simulink model "Dynamic_RR"  (R2019b)
settings: Solver=VariableStepAuto  StartTime=0.0  StopTime=30  FixedStep=1e-2  RelTol=1e-3
undefined symbols (not defined in the file): pi_hat_0, pi_param, qInitial_0
settings Model: Creator=Stefano  LastModifiedBy=Stefano

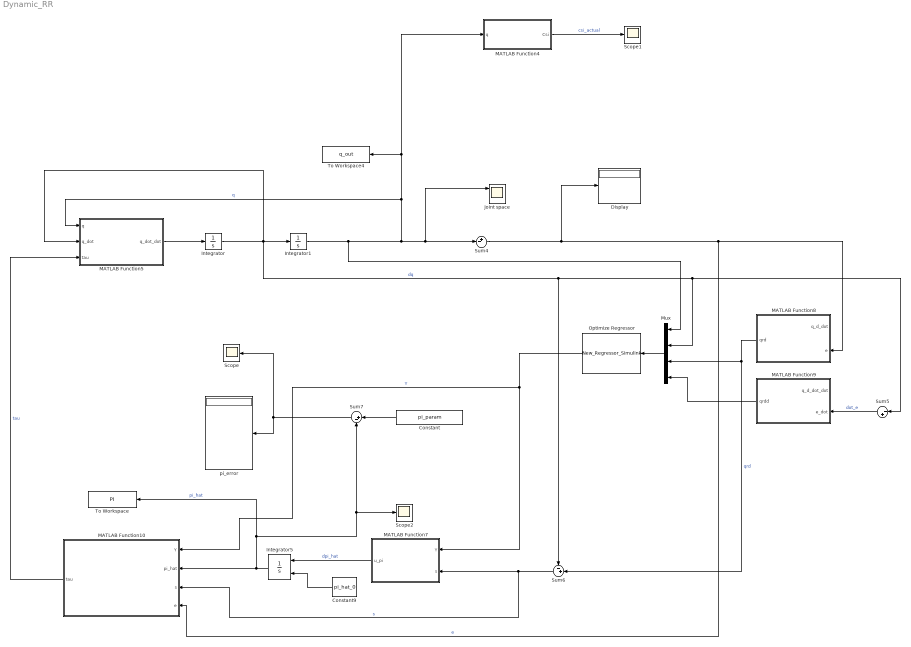
== system Dynamic_RR ==
  Constant : Constant  Value=pi_param
  Constant9 : Constant  Value=pi_hat_0
  Display : Display
  Integrator : Integrator  InitialCondition=qInitial_0
  Integrator1 : Integrator  InitialCondition=[0,0]'
  Integrator5 : Integrator  InitialConditionSource=external
  Joint space : Scope  NumInputPorts=2
  MATLAB Function10 : MATLAB Function  TreatAsAtomicUnit=on
  MATLAB Function4 : MATLAB Function  TreatAsAtomicUnit=on
  MATLAB Function5 : MATLAB Function  TreatAsAtomicUnit=on
  MATLAB Function7 : MATLAB Function  TreatAsAtomicUnit=on
  MATLAB Function8 : MATLAB Function  TreatAsAtomicUnit=on
  MATLAB Function9 : MATLAB Function  TreatAsAtomicUnit=on
  Mux : Mux
  "Optimize Regressor " : MATLABFcn  MATLABFcn=New_Regressor_Simulink  OutputDimensions=[2,6]  Output1D=off
  Scope : Scope
  Scope1 : Scope
  Scope2 : Scope
  Sum4 : Sum  Inputs=+-|
  Sum5 : Sum  Inputs=|-+
  Sum6 : Sum  Inputs=-+|
  Sum7 : Sum  Inputs=|+-
  To Workspace : ToWorkspace  VariableName=PI  SaveFormat=Timeseries  SampleTime=-1
  To Workspace4 : ToWorkspace  VariableName=q_out  SaveFormat=Timeseries  SampleTime=-1
  pi_error : Display
  wires:
  Sum6/1 -> MATLAB Function10/3(s), MATLAB Function7/2(s)  "s"
  Sum4/1 -> Display/1, MATLAB Function10/4(e), MATLAB Function8/2(e)  "e"
  Sum5/1 -> MATLAB Function9/2(e_dot)  "dot_e"
  MATLAB Function7/1(u_pi) -> Integrator5/1  "dpi_hat"
  Integrator5/1 -> MATLAB Function10/2(pi_hat), To Workspace/1, Scope2/1, Sum7/2  "pi_hat"
  Integrator/1 -> MATLAB Function5/2(q_dot), Sum5/1, Mux/2, Sum6/1, Integrator1/1  "dq"
  Constant9/1 -> Integrator5/2
  MATLAB Function8/1(qrd) -> Sum6/2, Mux/3  "qrd"
  Mux/1 -> "Optimize Regressor "/1
  MATLAB Function9/1(qrdd) -> Mux/4
  Constant/1 -> Sum7/1
  Sum7/1 -> Scope/1, pi_error/1
  Integrator1/1 -> Mux/1, To Workspace4/1, MATLAB Function4/1(q), MATLAB Function5/1(q), Joint space/1, Sum4/2  "q"
  "Optimize Regressor "/1 -> MATLAB Function10/1(Y), MATLAB Function7/1(Y)  "Y"
  MATLAB Function10/1(tau) -> MATLAB Function5/3(tau)  "tau"
  MATLAB Function5/1(q_dot_dot) -> Integrator/1
  ? -> Joint space/2, Sum4/1
  ? -> MATLAB Function8/1(q_d_dot), Sum5/2
  ? -> MATLAB Function9/1(q_d_dot_dot)
  MATLAB Function4/1(Csi) -> Scope1/1  "csi_actual"

== matlab function Dynamic_RR/MATLAB Function5 ==
  data: q input; q_dot_dot output; q_dot input; tau input
function q_dot_dot = Forward_Dynamics(q,q_dot,tau)

m1 = 1;
m2 = 1;

l1=1;
l2=1;

r1=l1/2;
r2=l2/2;


Izz1 = (1/12)*m1*l1^2;
Izz2 = (1/12)*m2*l2^2;



Alpha = Izz1 + Izz2 + m1*(r1)^2 + m2*(l1^2+r2^2);
Beta = m2*l1*r2;
Delta = Izz2 +m2*r2^2;

M = [Alpha + 2* Beta *cos(q(2)), Delta + Beta *cos(q(2));
     Delta + Beta *cos(q(2)),    Delta];

C = [-Beta*sin(q(2))*q_dot(2), -Beta*sin(q(2))*(q_dot(1)+q_dot(2));
     Beta*sin(q(2))*q_dot(1),   0];



q_dot_dot = inv(M)*([tau(1); tau(2)]- C*[q_dot(1); q_dot(2)]);

== matlab function Dynamic_RR/MATLAB Function4 ==
  data: q input; Csi output
function Csi  = Direct_Kinematics_RR(q)

%INPUT: q(1) = q1;
%       q(2) = q2;

%OUTPUT: px = position along x axis
%        py = position along y axis

%Link's lenght

l1 = 1;
l2 = 1;

px = l1 * cos(q(1)) + l2 * cos(q(1)+q(2));
py = l1 * sin(q(1)) + l2 * sin(q(1)+q(2));

Csi = [px; py];
end

== matlab function Dynamic_RR/MATLAB Function10 ==
  data: Y input; tau output; pi_hat input; s input; e input
function tau = Back_Stepping_Control_Law(Y,pi_hat,s,e)

Kd = 10 * eye(2);
Kp = 10 * eye(2);

tau = Y * pi_hat + Kd * s + Kp * e;

end

== matlab function Dynamic_RR/MATLAB Function7 ==
  data: Y input; u_pi output; s input
function u_pi = Update_Law(Y,s)

R = eye(2,4);
u_pi = pinv(R).*(Y.')*s;
end

== matlab function Dynamic_RR/MATLAB Function8 ==
  data: q_d_dot input; qrd output; e input
function qrd = q_r_dot(q_d_dot,e)

lambda = 7  * eye(2);
qrd = q_d_dot + lambda * e;

end

== matlab function Dynamic_RR/MATLAB Function9 ==
  data: q_d_dot_dot input; qrdd output; e_dot input
function qrdd = q_r_dot_dot(q_d_dot_dot,e_dot)

lambda = 7 * eye(2);
qrdd = q_d_dot_dot + lambda*e_dot;

end
